simulink model "PLL_example"  (R2020a)
settings: Solver=ode23  StartTime=0.0  StopTime=4e-6  MaxStep=1e-11  RelTol=1e-3  EnableMultiTasking=on
libraries: simulink x4
settings Model: Creator=Tony  LastModifiedBy=Tony
settings DataIOCC: LimitDataPoints=on  SaveFormat=Array  SignalLoggingSaveFormat=ModelDataLogs  ReturnWorkspaceOutputs=off
settings OptimizationCC: ExpressionDepthLimit=2147483647  InitFltsAndDblsToZero=on  LifeSpan=inf
settings DebuggingCC: SaveWithParameterizedLinksMsg=none  UnderspecifiedInitializationDetection=Classic  MergeDetectMultiDrivingBlocksExec=none  SignalResolutionControl=TryResolveAllWithWarning  SolverPrmCheckMsg=warning  MultiTaskDSMMsg=warning  MultiTaskCondExecSysMsg=none  FcnCallInpInsideContextMsg=warning  StateNameClashWarn=warning  SFUnexpectedBacktrackingDiag=warning  SFNoUnconditionalDefaultTransitionDiag=warning  SFExecutionAtInitializationDiag=none  ArithmeticOperatorsInVariantConditions=warning
settings HardwareCC: ProdBitPerPointer=32  ProdBitPerSizeT=32  ProdBitPerPtrDiffT=32  ProdLargestAtomicFloat=None  ProdIntDivRoundTo=Undefined  ProdEndianess=Unspecified  ProdWordSize=32  ProdHWDeviceType=32-bit Generic
settings ModelReferenceCC: PropagateSignalLabelsOutOfModel=off
settings SFSimCC: SimUseLocalCustomCode=off  CustomCodeUndefinedFunction=UseInterfaceOnly
settings RTWCC: RTWUseLocalCustomCode=off
settings CodeAppCC: StateflowObjectComments=on
settings GRTTargetCC: TargetFcnLib=ansi_tfl_tmw.mat  TargetLangStandard=C89/C90 (ANSI)  CombineOutputUpdateFcns=off  GRTInterface=on
settings ConfigComp: CovMetricSettings=dw  CovHtmlReporting=on  CovSaveCumulativeToWorkspaceVar=on  CovSaveSingleToWorkspaceVar=on  CovExternalEMLEnable=off

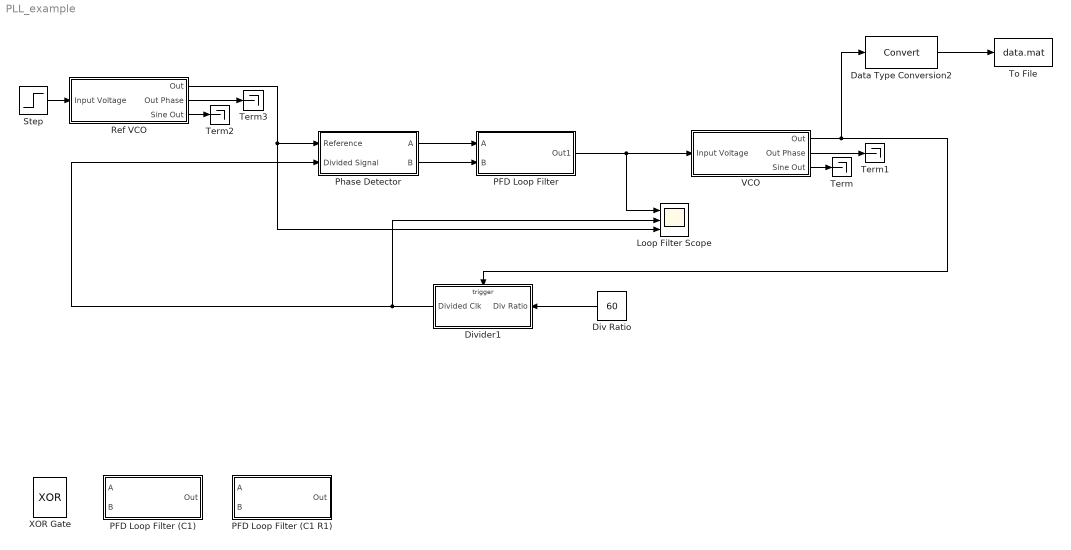
== system PLL_example ==
  Data Type Conversion2 : DataTypeConversion
  Div Ratio : Constant  Value=60  OutDataTypeStr=int32
  Divider1 : Subsystem
  Loop Filter Scope : Scope  NumInputPorts=3
  PFD Loop Filter : Subsystem  mask{Iu=25e-6, Id=25e-6, R1=6400, C1=16e-12, C2=1.6e-12}
      mask prompts: Iu "Loop Filter Pull Up Current (Iu)"; Id "Loop Filter Pull Down Current (Id)"
  PFD Loop Filter (C1 R1) : Subsystem  mask{Iu=25e-6, Id=25e-6, R1=8400, C1=16e-12}
      mask prompts: Iu "Loop Filter Pull Up Current (Iu)"; Id "Loop Filter Pull Down Current (Id)"
  PFD Loop Filter (C1) : Subsystem  mask{Iu=25e-6, Id=25e-6, C1=16e-12}
      mask prompts: Iu "Loop Filter Pull Up Current (Iu)"; Id "Loop Filter Pull Down Current (Id)"
  Phase Detector : Subsystem
  Ref VCO : Subsystem  mask{Kvco=20e6*2*pi, Ac=1, fo=0}
      mask prompts: fo "Default Frequency (fo)"
  Step : Step  Time=0  SampleTime=0
  Term{,1..3} (4 alike) : Terminator
  To File : ToFile  Filename=data.mat
  VCO : Subsystem  mask{Kvco=1e9*2*pi, Ac=1, fo=1000e6}
      mask prompts: fo "Default Frequency (fo)"
  XOR Gate : Logic  Operator=XOR  AllPortsSameDT=off  OutDataTypeStr=boolean
  wires:
  Divider1/1(Divided Clk) -> Phase Detector/2(Divided Signal), Loop Filter Scope/2
  VCO/1(Out) -> Data Type Conversion2/1, Divider1/Trigger
  Phase Detector/1(A) -> PFD Loop Filter/1(A)
  Phase Detector/2(B) -> PFD Loop Filter/2(B)
  PFD Loop Filter/1(Out1) -> VCO/1(Input Voltage), Loop Filter Scope/1
  Data Type Conversion2/1 -> To File/1
  Ref VCO/1(Out) -> Phase Detector/1(Reference), Loop Filter Scope/3
  Step/1 -> Ref VCO/1(Input Voltage)
  Div Ratio/1 -> Divider1/1(Div Ratio)
  VCO/3(Sine Out) -> Term/1
  VCO/2(Out Phase) -> Term1/1
  Ref VCO/3(Sine Out) -> Term2/1
  Ref VCO/2(Out Phase) -> Term3/1

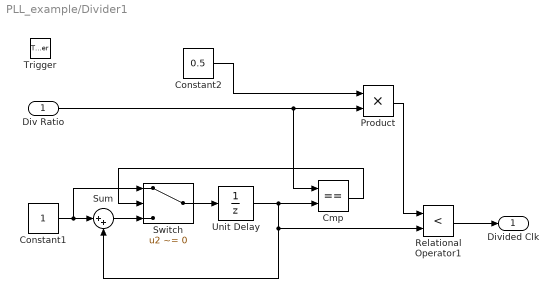
== system PLL_example/Divider1 ==
  Div Ratio : Inport
  Trigger : TriggerPort  VariantControl=(inherit)
  Cmp : RelationalOperator  Operator===  OutDataTypeStr=boolean  RndMeth=Nearest
  Constant1 : Constant  OutDataTypeStr=int32
  Constant2 : Constant  Value=0.5
  Product : Product  RndMeth=Zero
  Relational Operator1 : RelationalOperator  Operator=<  OutDataTypeStr=boolean  RndMeth=Nearest
  Sum : Sum  Inputs=|++
  Switch : Switch  Criteria=u2 ~= 0
  Unit Delay : UnitDelay  SampleTime=-1
  Divided Clk : Outport
  wires:
  Constant1/1 -> Sum/1, Switch/1
  Sum/1 -> Switch/3
  Cmp/1 -> Switch/2
  Div Ratio/1 -> Cmp/1, Product/2
  Constant2/1 -> Product/1
  Product/1 -> Relational Operator1/1
  Relational Operator1/1 -> Divided Clk/1
  Unit Delay/1 -> Cmp/2, Relational Operator1/2, Sum/2
  Switch/1 -> Unit Delay/1

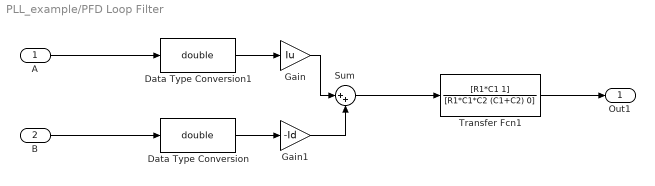
== system PLL_example/PFD Loop Filter ==
  A : Inport
  B : Inport  Port=2
  Data Type Conversion : DataTypeConversion  OutDataTypeStr=double
  Data Type Conversion1 : DataTypeConversion  OutDataTypeStr=double
  Gain : Gain  Gain=Iu
  Gain1 : Gain  Gain=-Id
  Sum : Sum  Inputs=|++
  Transfer Fcn1 : TransferFcn  Numerator=[R1*C1 1]  Denominator=[R1*C1*C2 (C1+C2) 0]
  Out1 : Outport
  wires:
  Data Type Conversion1/1 -> Gain/1
  Gain/1 -> Sum/1
  Data Type Conversion/1 -> Gain1/1
  Gain1/1 -> Sum/2
  Sum/1 -> Transfer Fcn1/1
  Transfer Fcn1/1 -> Out1/1
  B/1 -> Data Type Conversion/1
  A/1 -> Data Type Conversion1/1

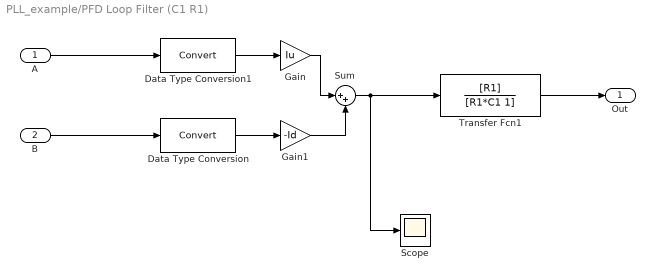
== system PLL_example/PFD Loop Filter (C1 R1) ==
  A : Inport
  B : Inport  Port=2
  Data Type Conversion : DataTypeConversion
  Data Type Conversion1 : DataTypeConversion
  Gain : Gain  Gain=Iu
  Gain1 : Gain  Gain=-Id
  Scope : Scope
  Sum : Sum  Inputs=|++
  Transfer Fcn1 : TransferFcn  Numerator=[R1]  Denominator=[R1*C1 1]
  Out : Outport
  wires:
  Data Type Conversion1/1 -> Gain/1
  Gain/1 -> Sum/1
  Data Type Conversion/1 -> Gain1/1
  Gain1/1 -> Sum/2
  Sum/1 -> Scope/1, Transfer Fcn1/1
  Transfer Fcn1/1 -> Out/1
  B/1 -> Data Type Conversion/1
  A/1 -> Data Type Conversion1/1

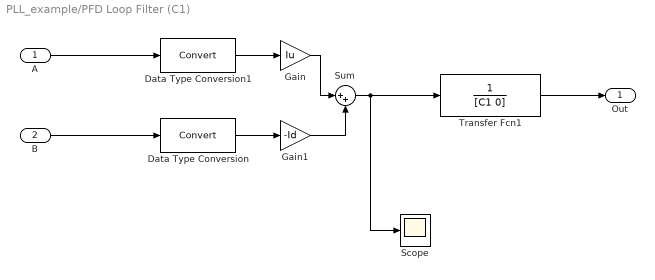
== system PLL_example/PFD Loop Filter (C1) ==
  A : Inport
  B : Inport  Port=2
  Data Type Conversion : DataTypeConversion
  Data Type Conversion1 : DataTypeConversion
  Gain : Gain  Gain=Iu
  Gain1 : Gain  Gain=-Id
  Scope : Scope
  Sum : Sum  Inputs=|++
  Transfer Fcn1 : TransferFcn  Denominator=[C1 0]
  Out : Outport
  wires:
  Data Type Conversion1/1 -> Gain/1
  Gain/1 -> Sum/1
  Data Type Conversion/1 -> Gain1/1
  Gain1/1 -> Sum/2
  Sum/1 -> Scope/1, Transfer Fcn1/1
  Transfer Fcn1/1 -> Out/1
  B/1 -> Data Type Conversion/1
  A/1 -> Data Type Conversion1/1

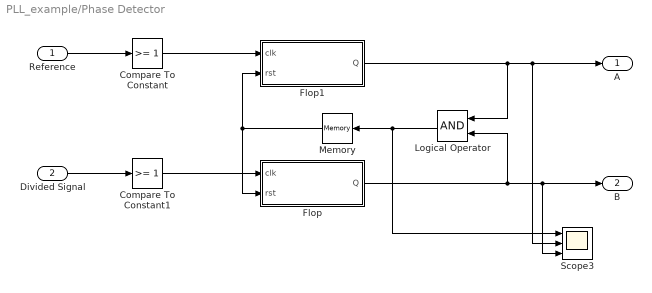
== system PLL_example/Phase Detector ==
  Reference : Inport
  Divided Signal : Inport  Port=2
  Compare To Constant : simulink/Logic and Bit Operations/Compare To Constant  relop=>=  const=1  OutDataTypeStr=boolean  ZeroCross=off
  Compare To Constant1 : simulink/Logic and Bit Operations/Compare To Constant  relop=>=  const=1  OutDataTypeStr=boolean  ZeroCross=off
  Flop : Subsystem
  Flop1 : Subsystem
  Logical Operator : Logic  AllPortsSameDT=off  OutDataTypeStr=boolean
  Memory : Memory
  Scope3 : Scope  NumInputPorts=3
  A : Outport
  B : Outport  Port=2
  wires:
  Flop1/1(Q) -> Logical Operator/1, A/1, Scope3/2
  Flop/1(Q) -> Logical Operator/2, B/1, Scope3/3
  Reference/1 -> Compare To Constant/1
  Compare To Constant/1 -> Flop1/1(clk)
  Divided Signal/1 -> Compare To Constant1/1
  Compare To Constant1/1 -> Flop/1(clk)
  Logical Operator/1 -> Scope3/1, Memory/1
  Memory/1 -> Flop/2(rst), Flop1/2(rst)

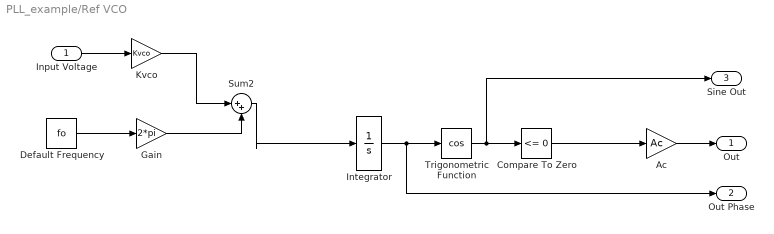
== system PLL_example/Ref VCO ==
  Input Voltage : Inport
  Ac : Gain  Gain=Ac
  Compare To Zero : simulink/Logic and Bit Operations/Compare To Zero  relop=<=  OutDataTypeStr=uint8
  Default Frequency : Constant  Value=fo
  Gain : Gain  Gain=2*pi
  Integrator : Integrator
  Kvco : Gain  Gain=Kvco
  Sum2 : Sum  Inputs=|++
  Trigonometric Function : Trigonometry  Operator=cos
  Out : Outport
  Out Phase : Outport  Port=2
  Sine Out : Outport  Port=3
  wires:
  Ac/1 -> Out/1
  Compare To Zero/1 -> Ac/1
  Trigonometric Function/1 -> Sine Out/1, Compare To Zero/1
  Default Frequency/1 -> Gain/1
  Input Voltage/1 -> Kvco/1
  Integrator/1 -> Out Phase/1, Trigonometric Function/1
  Sum2/1 -> Integrator/1
  Gain/1 -> Sum2/2
  Kvco/1 -> Sum2/1

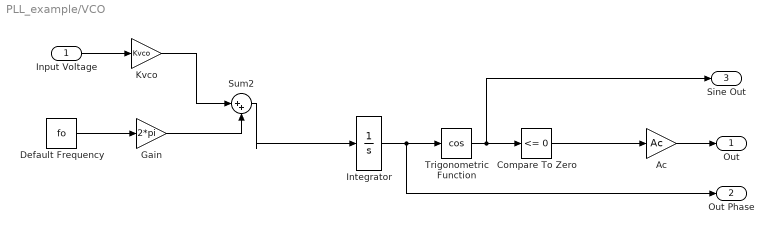
== system PLL_example/VCO ==
  Input Voltage : Inport
  Ac : Gain  Gain=Ac
  Compare To Zero : simulink/Logic and Bit Operations/Compare To Zero  relop=<=  OutDataTypeStr=uint8
  Default Frequency : Constant  Value=fo
  Gain : Gain  Gain=2*pi
  Integrator : Integrator
  Kvco : Gain  Gain=Kvco  OutDataTypeStr=Inherit: Inherit via back propagation
  Sum2 : Sum  Inputs=|++
  Trigonometric Function : Trigonometry  Operator=cos
  Out : Outport
  Out Phase : Outport  Port=2
  Sine Out : Outport  Port=3
  wires:
  Kvco/1 -> Sum2/1
  Gain/1 -> Sum2/2
  Sum2/1 -> Integrator/1
  Integrator/1 -> Trigonometric Function/1, Out Phase/1
  Input Voltage/1 -> Kvco/1
  Default Frequency/1 -> Gain/1
  Trigonometric Function/1 -> Compare To Zero/1, Sine Out/1
  Compare To Zero/1 -> Ac/1
  Ac/1 -> Out/1

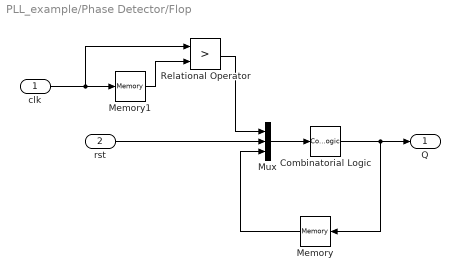
== system PLL_example/Phase Detector/Flop ==
  clk : Inport
  rst : Inport  Port=2
  Combinatorial Logic : CombinatorialLogic  TruthTable=[0;1;0;0;1;1;0;0]
  Memory : Memory
  Memory1 : Memory
  Mux : Mux  Inputs=3
  Relational Operator : RelationalOperator  Operator=>  OutDataTypeStr=boolean  RndMeth=Nearest
  Q : Outport
  wires:
  Mux/1 -> Combinatorial Logic/1
  rst/1 -> Mux/2
  Combinatorial Logic/1 -> Memory/1, Q/1
  Memory/1 -> Mux/3
  clk/1 -> Relational Operator/1, Memory1/1
  Memory1/1 -> Relational Operator/2
  Relational Operator/1 -> Mux/1

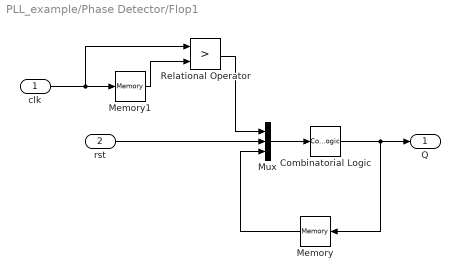
== system PLL_example/Phase Detector/Flop1 ==
  clk : Inport
  rst : Inport  Port=2
  Combinatorial Logic : CombinatorialLogic  TruthTable=[0;1;0;0;1;1;0;0]
  Memory : Memory
  Memory1 : Memory
  Mux : Mux  Inputs=3
  Relational Operator : RelationalOperator  Operator=>  OutDataTypeStr=boolean  RndMeth=Nearest
  Q : Outport
  wires:
  Mux/1 -> Combinatorial Logic/1
  rst/1 -> Mux/2
  Combinatorial Logic/1 -> Q/1, Memory/1
  Memory/1 -> Mux/3
  clk/1 -> Relational Operator/1, Memory1/1
  Memory1/1 -> Relational Operator/2
  Relational Operator/1 -> Mux/1
